simulink model "PID_Controller"  (R2020a)
settings: Solver=VariableStepAuto  StartTime=0.0  StopTime=120  RelTol=1e-3
values from neighbouring files (symbols this model uses):
  Kd = -165.0    [DD23.sldd]
  Ki = 28.0    [DD23.sldd]
  Kp = 254.0    [DD23.sldd]
settings Model: DataDictionary=DD23.sldd  Creator=HP  LastModifiedBy=HP
settings DataIOCC: SaveOutput=off  SaveTime=off

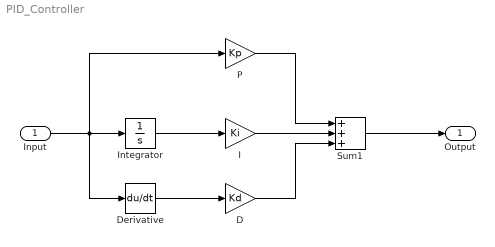
== system PID_Controller ==
  Input : Inport  OutDataTypeStr=double  PortDimensions=1  SampleTime=0
  D : Gain  Gain=Kd
  Derivative : Derivative
  I : Gain  Gain=Ki
  Integrator : Integrator
  P : Gain  Gain=Kp
  Sum1 : Sum  Inputs=+++
  Output : Outport  OutDataTypeStr=double  PortDimensions=1  SampleTime=0
  wires:
  Input/1 -> P/1, Integrator/1, Derivative/1
  Sum1/1 -> Output/1
  I/1 -> Sum1/2
  P/1 -> Sum1/1
  Integrator/1 -> I/1
  Derivative/1 -> D/1
  D/1 -> Sum1/3
